simulink model "gm_waveMulTest"  (R2023b)
settings: Solver=VariableStepAuto  StartTime=0.0  StopTime=10000/fs  RelTol=1e-3
undefined symbols (not defined in the file or in its folder): fs, inputData, num
libraries: dsphdlsigops2 x1, hdlsllib x1
settings Model: Creator=31651  LastModifiedBy=31651
settings OptimizationCC: BlockReduction=off  ConditionallyExecuteInputs=off
settings DebuggingCC: InheritedTsInSrcMsg=none

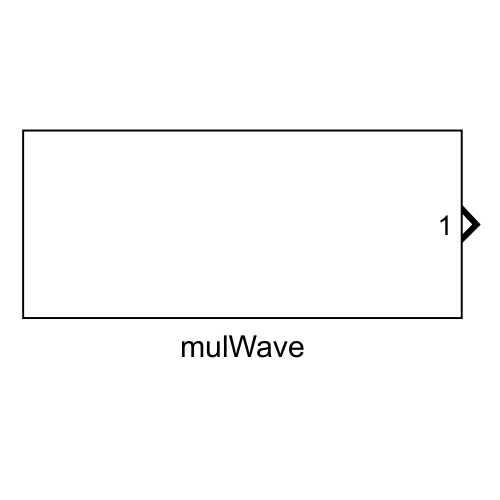
[thumbnail: Simulink's stored preview of the top-level diagram]
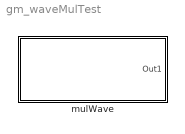
== system gm_waveMulTest ==
  mulWave : Subsystem

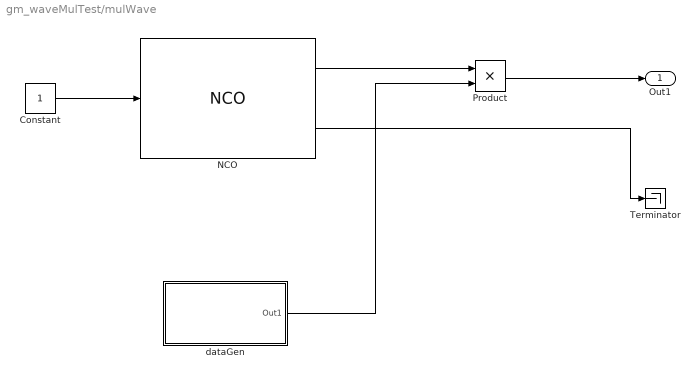
== system gm_waveMulTest/mulWave ==
  Constant : Constant  OutDataTypeStr=boolean  SampleTime=1/fs
  NCO : dsphdlsigops2/NCO  PhaseIncrementSource=Property  PhaseIncrement=phInc  PhaseOffsetSource=Property  PhaseOffset=0  DitherSource=Property  NumDitherBits=4  SamplesPerFrame=1  LUTCompress=off  ResetAction=off  Waveform=Sine  PhasePort=off  SimulateUsing=Code generation  AccumulatorWL=N  PhaseQuantization=on  NumQuantizerAccumulatorBits=Q  OutputDataType=Binary point scaling  OutputWL=16  OutputFL=14
      settings: LibrarySourceBlock=dsphdlsrcs2/NCO
  Product : Product
  Terminator : Terminator
  dataGen : Subsystem
  Out1 : Outport
  wires:
  dataGen/1(Out1) -> Product/2
  NCO/2 -> Terminator/1
  Product/1 -> Out1/1
  NCO/1 -> Product/1
  Constant/1 -> NCO/1

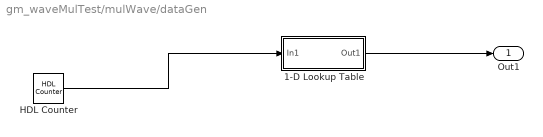
== system gm_waveMulTest/mulWave/dataGen ==
  1-D Lookup Table : Subsystem
  HDL Counter : hdlsllib/Sources/HDL Counter  CountType=Count limited  CountInit=0  CountStep=1  CountMax=2*num-1  CountFromType=Initial value  CountFrom=0  CountResetPort=off  CountLoadPort=off  CountEnbPort=off  CountDirPort=off  CountHitOutputPort=off  CountDataType=Unsigned  CountWordLen=8  CountFracLen=0  CountSampTime=1/fs
  Out1 : Outport  OutDataTypeStr=int8  SampleTime=1e-08
  wires:
  1-D Lookup Table/1(Out1) -> Out1/1
  HDL Counter/1 -> 1-D Lookup Table/1(In1)

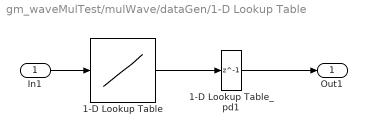
== system gm_waveMulTest/mulWave/dataGen/1-D Lookup Table ==
  In1 : Inport
  1-D Lookup Table : Lookup_n-D  NumberOfTableDimensions=1  LookupTableObject=''  BreakpointsForDimension1=[0:2*num-1]  BreakpointsForDimension1FirstPoint=10  BreakpointsForDimension2FirstPoint=10  BreakpointsForDimension1Spacing=12  BreakpointsForDimension2Spacing=12  IndexSearchMethod=Evenly spaced points  Table=inputData  InterpMethod=Flat  InternalRulePriority=Speed  OutDataTypeStr=int8  RndMeth=Simplest
  1-D Lookup Table_pd1 : Delay  DelayLength=1
  Out1 : Outport
  wires:
  In1/1 -> 1-D Lookup Table/1
  1-D Lookup Table/1 -> 1-D Lookup Table_pd1/1
  1-D Lookup Table_pd1/1 -> Out1/1
